simulink model "SwitchMobility_ACC"  (R2022b)
settings: Solver=ode1  StartTime=0.0  StopTime=inf  FixedStep=0.001  RelTol=1e-3
PreLoadFcn:
  | vehicle = 'Truck'; if ~length(which('cmself')), cmenv; end
  | SwitchMobility_ACC_bus
InitFcn:
  | vehicle = 'Truck'; if ~length(which('cmself')), cmenv; end
  | SwitchMobility_ACC_bus
libraries: CarMaker4SL x32, simulink x1
Description:
  | CarMaker Plug-in Model Target
settings Model: Creator=satyaprakash.gupta  LastModifiedBy=satyaprakash.gupta
settings RTWCC: Description=CarMaker Plug-in Model Target  SystemTargetFile=CarMaker.tlc  TemplateMakefile=CarMaker_unix-win64.tmf
settings CodeAppCC: MaxIdLength=127
settings STFCustomTargetCC: TargetLangStandard=C99 (ISO)  CombineOutputUpdateFcns=on  CodeInterfacePackaging=Reusable function  GenerateAllocFcn=on  SystemTargetFile=CarMaker.tlc
settings GRTTargetCC: ParMdlRefBuildCompliant=off  CompOptLevelCompliant=off  ConcurrentExecutionCompliant=off  MatFileLogging=off  CodeInterfacePackaging=Reusable function  CPPClassGenCompliant=off  GenerateAllocFcn=on  UseToolchainInfoCompliant=off

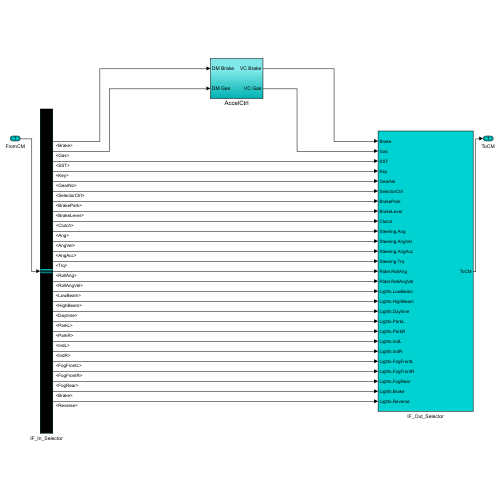
[thumbnail: Simulink's stored preview of the top-level diagram]
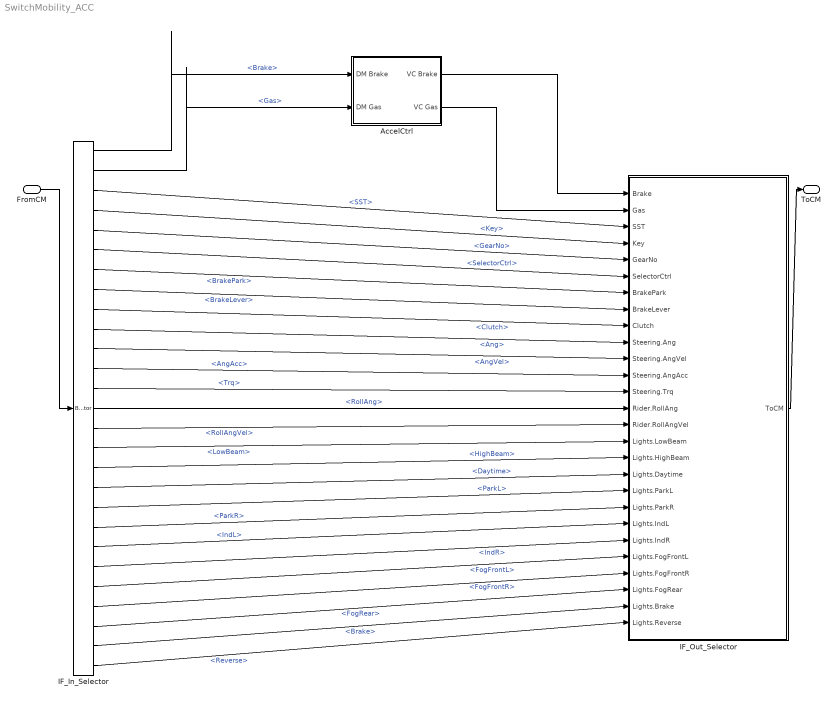
== system SwitchMobility_ACC ==
  FromCM : Inport  OutDataTypeStr=Bus: cmVehicleControlIn
  AccelCtrl : Subsystem
  IF_In_Selector : BusSelector  OutputSignals=Brake,Gas,SST,Key,GearNo,SelectorCtrl,BrakePark,BrakeLever,Clutch,Steering.Ang,Steering.AngVel,Steering.AngAcc,Steering.Trq,Rider.RollAng,Rider.RollAngVel,Lights.LowBeam,Lights.HighBeam,Lights.Daytime,Lights.ParkL,Lights.ParkR,Lights.IndL,Lights.IndR,Lights.FogFrontL,Lights.FogFrontR,Lights.FogRear,Lights.Brake,Lights.Reverse
  IF_Out_Selector : Subsystem  mask(Signal Selection){}
      mask help: Signal Selection Block
      settings: OpenFcn=cmSignalSelect('SignalSelection_CB',gcb)
  ToCM : Outport  OutDataTypeStr=Bus: cmVehicleControlOut
  wires:
  FromCM/1 -> IF_In_Selector/1
  IF_In_Selector/1 -> AccelCtrl/1(DM Brake)  "<Brake>"
  IF_Out_Selector/1(ToCM) -> ToCM/1
  AccelCtrl/1(VC Brake) -> IF_Out_Selector/1(Brake)
  AccelCtrl/2(VC Gas) -> IF_Out_Selector/2(Gas)
  IF_In_Selector/2 -> AccelCtrl/2(DM Gas)  "<Gas>"
  IF_In_Selector/3 -> IF_Out_Selector/3(SST)  "<SST>"
  IF_In_Selector/4 -> IF_Out_Selector/4(Key)  "<Key>"
  IF_In_Selector/5 -> IF_Out_Selector/5(GearNo)  "<GearNo>"
  IF_In_Selector/6 -> IF_Out_Selector/6(SelectorCtrl)  "<SelectorCtrl>"
  IF_In_Selector/7 -> IF_Out_Selector/7(BrakePark)  "<BrakePark>"
  IF_In_Selector/8 -> IF_Out_Selector/8(BrakeLever)  "<BrakeLever>"
  IF_In_Selector/9 -> IF_Out_Selector/9(Clutch)  "<Clutch>"
  IF_In_Selector/10 -> IF_Out_Selector/10(Steering.Ang)  "<Ang>"
  IF_In_Selector/11 -> IF_Out_Selector/11(Steering.AngVel)  "<AngVel>"
  IF_In_Selector/12 -> IF_Out_Selector/12(Steering.AngAcc)  "<AngAcc>"
  IF_In_Selector/13 -> IF_Out_Selector/13(Steering.Trq)  "<Trq>"
  IF_In_Selector/14 -> IF_Out_Selector/14(Rider.RollAng)  "<RollAng>"
  IF_In_Selector/15 -> IF_Out_Selector/15(Rider.RollAngVel)  "<RollAngVel>"
  IF_In_Selector/16 -> IF_Out_Selector/16(Lights.LowBeam)  "<LowBeam>"
  IF_In_Selector/17 -> IF_Out_Selector/17(Lights.HighBeam)  "<HighBeam>"
  IF_In_Selector/18 -> IF_Out_Selector/18(Lights.Daytime)  "<Daytime>"
  IF_In_Selector/19 -> IF_Out_Selector/19(Lights.ParkL)  "<ParkL>"
  IF_In_Selector/20 -> IF_Out_Selector/20(Lights.ParkR)  "<ParkR>"
  IF_In_Selector/21 -> IF_Out_Selector/21(Lights.IndL)  "<IndL>"
  IF_In_Selector/22 -> IF_Out_Selector/22(Lights.IndR)  "<IndR>"
  IF_In_Selector/23 -> IF_Out_Selector/23(Lights.FogFrontL)  "<FogFrontL>"
  IF_In_Selector/24 -> IF_Out_Selector/24(Lights.FogFrontR)  "<FogFrontR>"
  IF_In_Selector/25 -> IF_Out_Selector/25(Lights.FogRear)  "<FogRear>"
  IF_In_Selector/26 -> IF_Out_Selector/26(Lights.Brake)  "<Brake>"
  IF_In_Selector/27 -> IF_Out_Selector/27(Lights.Reverse)  "<Reverse>"

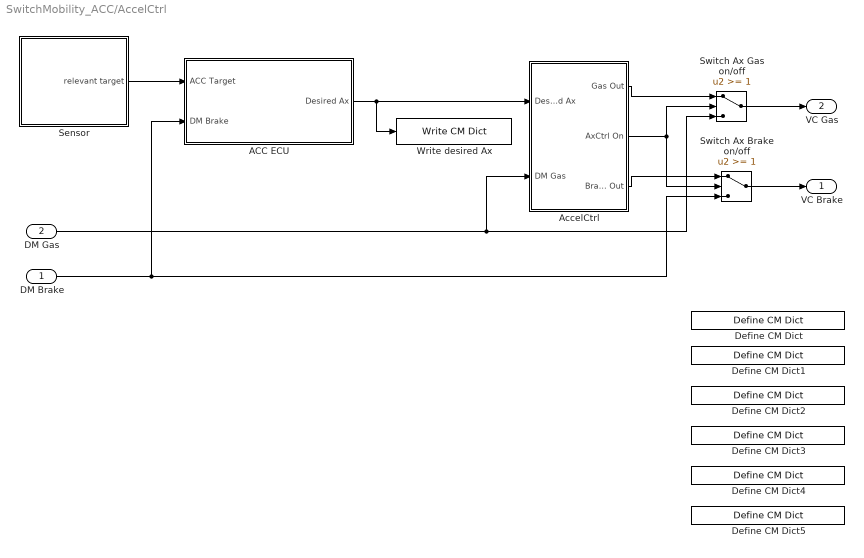
== system SwitchMobility_ACC/AccelCtrl ==
  DM Brake : Inport
  DM Gas : Inport  Port=2
  ACC ECU : Subsystem
  AccelCtrl : Subsystem
  Define CM Dict : CarMaker4SL/Define CM Dict  xname=AccelCtrl.ACC.IsActive  xmono=off  xtype=Char  xdvaplace=DM  xnstates=2  xfirststate=0  xinitial=1
  Define CM Dict1 : CarMaker4SL/Define CM Dict  xname=AccelCtrl.ACC.DesiredTGap  xunit=s  xmono=off  xtype=Double4  xdvaplace=DM  xnstates=0  xfirststate=0  xinitial=0
  Define CM Dict2 : CarMaker4SL/Define CM Dict  xname=AccelCtrl.ACC.DesiredSpd  xunit=m/s  xmono=off  xtype=Double4  xdvaplace=DM  xnstates=0  xfirststate=0  xinitial=0
  Define CM Dict3 : CarMaker4SL/Define CM Dict  xname=AccelCtrl.ACC.DesiredAx  xunit=m/s^2  xmono=off  xtype=Double4  xdvaplace=DM  xnstates=0  xfirststate=0  xinitial=0
  Define CM Dict4 : CarMaker4SL/Define CM Dict  xname=AccelCtrl.DesiredAx  xunit=m/s^2  xmono=off  xtype=Double4  xdvaplace=DM  xnstates=0  xfirststate=0  xinitial=0
  Define CM Dict5 : CarMaker4SL/Define CM Dict  xname=AccelCtrl.ACC.DesiredDist  xunit=m  xmono=off  xtype=Double4  xdvaplace=DM  xnstates=0  xfirststate=0  xinitial=0
  Sensor : Subsystem
  Switch Ax Brake on/off : Switch  Threshold=1  InputSameDT=off
  Switch Ax Gas on/off : Switch  Threshold=1  InputSameDT=off
  Write desired Ax : CarMaker4SL/Write CM Dict  xname=AccelCtrl.DesiredAx  xsync=off
  VC Brake : Outport  VectorParamsAs1DForOutWhenUnconnected=off
  VC Gas : Outport  Port=2  VectorParamsAs1DForOutWhenUnconnected=off
  wires:
  Sensor/1(relevant target) -> ACC ECU/1(ACC Target)
  DM Brake/1 -> Switch Ax Brake on/off/3, ACC ECU/2(DM Brake)
  Switch Ax Gas on/off/1 -> VC Gas/1
  Switch Ax Brake on/off/1 -> VC Brake/1
  AccelCtrl/1(Gas Out) -> Switch Ax Gas on/off/1
  AccelCtrl/3(Brake Out) -> Switch Ax Brake on/off/1
  ACC ECU/1(Desired Ax) -> AccelCtrl/1(Desired Ax), Write desired Ax/1
  DM Gas/1 -> Switch Ax Gas on/off/3, AccelCtrl/2(DM Gas)
  AccelCtrl/2(AxCtrl On) -> Switch Ax Gas on/off/2, Switch Ax Brake on/off/2

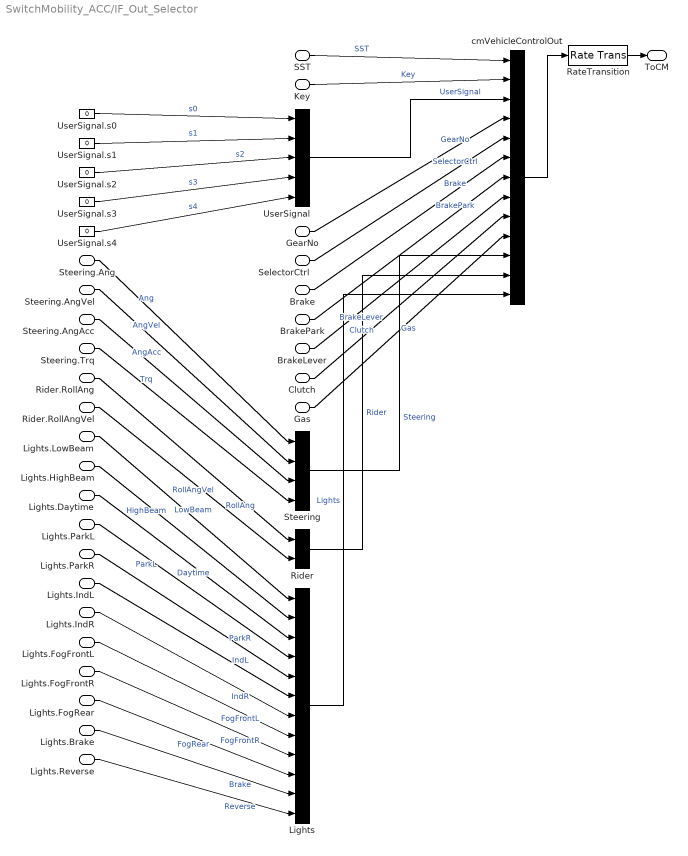
== system SwitchMobility_ACC/IF_Out_Selector ==
  Brake : Inport
  Gas : Inport  Port=2
  SST : Inport  Port=3
  Key : Inport  Port=4
  GearNo : Inport  Port=5
  SelectorCtrl : Inport  Port=6
  BrakePark : Inport  Port=7
  BrakeLever : Inport  Port=8
  Clutch : Inport  Port=9
  Steering.Ang : Inport  Port=10
  Steering.AngVel : Inport  Port=11
  Steering.AngAcc : Inport  Port=12
  Steering.Trq : Inport  Port=13
  Rider.RollAng : Inport  Port=14
  Rider.RollAngVel : Inport  Port=15
  Lights.LowBeam : Inport  Port=16
  Lights.HighBeam : Inport  Port=17
  Lights.Daytime : Inport  Port=18
  Lights.ParkL : Inport  Port=19
  Lights.ParkR : Inport  Port=20
  Lights.IndL : Inport  Port=21
  Lights.IndR : Inport  Port=22
  Lights.FogFrontL : Inport  Port=23
  Lights.FogFrontR : Inport  Port=24
  Lights.FogRear : Inport  Port=25
  Lights.Brake : Inport  Port=26
  Lights.Reverse : Inport  Port=27
  Lights : BusCreator  Inputs=12
  RateTransition : RateTransition  OutPortSampleTime=str2num(get_param(bdroot,'FixedStep'))
  Rider : BusCreator  Inputs=2
  Steering : BusCreator  Inputs=4
  UserSignal : BusCreator  Inputs=5
  UserSignal.s{0..4} (5 alike) : Constant  Value=0
  cmVehicleControlOut : BusCreator  Inputs=13
  ToCM : Outport
  wires:
  RateTransition/1 -> ToCM/1
  cmVehicleControlOut/1 -> RateTransition/1
  UserSignal/1 -> cmVehicleControlOut/3  "UserSignal"
  UserSignal.s0/1 -> UserSignal/1  "s0"
  UserSignal.s1/1 -> UserSignal/2  "s1"
  UserSignal.s2/1 -> UserSignal/3  "s2"
  UserSignal.s3/1 -> UserSignal/4  "s3"
  UserSignal.s4/1 -> UserSignal/5  "s4"
  Steering/1 -> cmVehicleControlOut/11  "Steering"
  Rider/1 -> cmVehicleControlOut/12  "Rider"
  Lights/1 -> cmVehicleControlOut/13  "Lights"
  Brake/1 -> cmVehicleControlOut/6  "Brake"
  Gas/1 -> cmVehicleControlOut/10  "Gas"
  SST/1 -> cmVehicleControlOut/1  "SST"
  Key/1 -> cmVehicleControlOut/2  "Key"
  GearNo/1 -> cmVehicleControlOut/4  "GearNo"
  SelectorCtrl/1 -> cmVehicleControlOut/5  "SelectorCtrl"
  BrakePark/1 -> cmVehicleControlOut/7  "BrakePark"
  BrakeLever/1 -> cmVehicleControlOut/8  "BrakeLever"
  Clutch/1 -> cmVehicleControlOut/9  "Clutch"
  Steering.Ang/1 -> Steering/1  "Ang"
  Steering.AngVel/1 -> Steering/2  "AngVel"
  Steering.AngAcc/1 -> Steering/3  "AngAcc"
  Steering.Trq/1 -> Steering/4  "Trq"
  Rider.RollAng/1 -> Rider/1  "RollAng"
  Rider.RollAngVel/1 -> Rider/2  "RollAngVel"
  Lights.LowBeam/1 -> Lights/1  "LowBeam"
  Lights.HighBeam/1 -> Lights/2  "HighBeam"
  Lights.Daytime/1 -> Lights/3  "Daytime"
  Lights.ParkL/1 -> Lights/4  "ParkL"
  Lights.ParkR/1 -> Lights/5  "ParkR"
  Lights.IndL/1 -> Lights/6  "IndL"
  Lights.IndR/1 -> Lights/7  "IndR"
  Lights.FogFrontL/1 -> Lights/8  "FogFrontL"
  Lights.FogFrontR/1 -> Lights/9  "FogFrontR"
  Lights.FogRear/1 -> Lights/10  "FogRear"
  Lights.Brake/1 -> Lights/11  "Brake"
  Lights.Reverse/1 -> Lights/12  "Reverse"

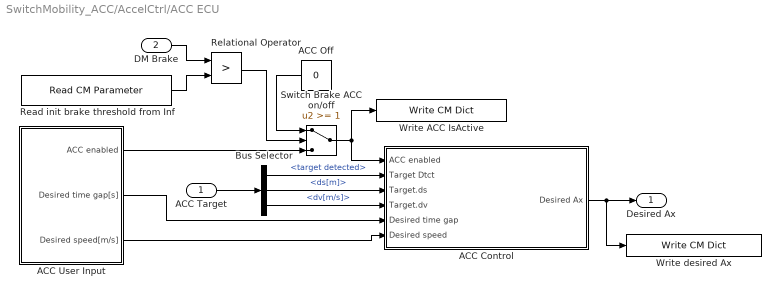
== system SwitchMobility_ACC/AccelCtrl/ACC ECU ==
  ACC Target : Inport
  DM Brake : Inport  Port=2
  ACC Control : Subsystem
  ACC Off : Constant  Value=0
  ACC User Input : Subsystem
  Bus Selector : BusSelector  OutputSignals=target detected,ds[m],dv[m/s]
  Read init brake threshold from Inf : CarMaker4SL/Read CM Parameter  xfile=Vehicle  xkey=AccelCtrl.ACC.BrakeThreshold  xnout=1  xdefaults=0.2  xmuxed=off  xstime=Continuous
      settings: SourceProductName=CarMaker4SL
  Relational Operator : RelationalOperator  Operator=>  InputSameDT=off
  Switch Brake ACC on/off : Switch  Threshold=1  InputSameDT=off
  Write ACC IsActive : CarMaker4SL/Write CM Dict  xname=AccelCtrl.ACC.IsActive  xsync=off
  Write desired Ax : CarMaker4SL/Write CM Dict  xname=AccelCtrl.ACC.DesiredAx  xsync=off
  Desired Ax : Outport  VectorParamsAs1DForOutWhenUnconnected=off
  wires:
  ACC Target/1 -> Bus Selector/1
  Bus Selector/2 -> ACC Control/3(Target.ds)  "<ds[m]>"
  Bus Selector/3 -> ACC Control/4(Target.dv)  "<dv[m/s]>"
  Bus Selector/1 -> ACC Control/2(Target Dtct)  "<target detected>"
  ACC Control/1(Desired Ax) -> Desired Ax/1, Write desired Ax/1
  ACC User Input/2(Desired time gap[s]) -> ACC Control/5(Desired time gap)
  ACC User Input/3(Desired speed[m/s]) -> ACC Control/6(Desired speed)
  DM Brake/1 -> Relational Operator/1
  ACC User Input/1(ACC enabled) -> Switch Brake ACC on/off/3
  Relational Operator/1 -> Switch Brake ACC on/off/2
  ACC Off/1 -> Switch Brake ACC on/off/1
  Switch Brake ACC on/off/1 -> ACC Control/1(ACC enabled), Write ACC IsActive/1
  Read init brake threshold from Inf/1 -> Relational Operator/2

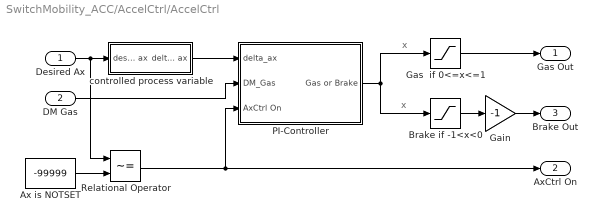
== system SwitchMobility_ACC/AccelCtrl/AccelCtrl ==
  note: x
  note: x
  Desired Ax : Inport
  DM Gas : Inport  Port=2
  Ax is NOTSET : Constant  Value=-99999
  Brake if -1<x<0 : Saturate  UpperLimit=0  LowerLimit=-1
  Gain : Gain  Gain=-1  SaturateOnIntegerOverflow=on  OutDataTypeStr=Inherit: Same as input  ParamDataTypeStr=Inherit: Same as input
  Gas  if 0<=x<=1 : Saturate  UpperLimit=1  LowerLimit=0
  PI-Controller : Subsystem
  Relational Operator : RelationalOperator  Operator=~=  InputSameDT=off
  "controlled process variable " : Subsystem
  Gas Out : Outport  VectorParamsAs1DForOutWhenUnconnected=off
  AxCtrl On : Outport  Port=2  VectorParamsAs1DForOutWhenUnconnected=off
  Brake Out : Outport  Port=3  VectorParamsAs1DForOutWhenUnconnected=off
  wires:
  Gain/1 -> Brake Out/1
  "controlled process variable "/1(delta ax) -> PI-Controller/1(delta_ax)
  DM Gas/1 -> PI-Controller/2(DM_Gas)
  Desired Ax/1 -> "controlled process variable "/1(desired ax), Relational Operator/1
  PI-Controller/1(Gas or Brake) -> Brake if -1<x<0/1, Gas  if 0<=x<=1/1
  Gas  if 0<=x<=1/1 -> Gas Out/1
  Brake if -1<x<0/1 -> Gain/1
  Ax is NOTSET/1 -> Relational Operator/2
  Relational Operator/1 -> AxCtrl On/1, PI-Controller/3(AxCtrl On)

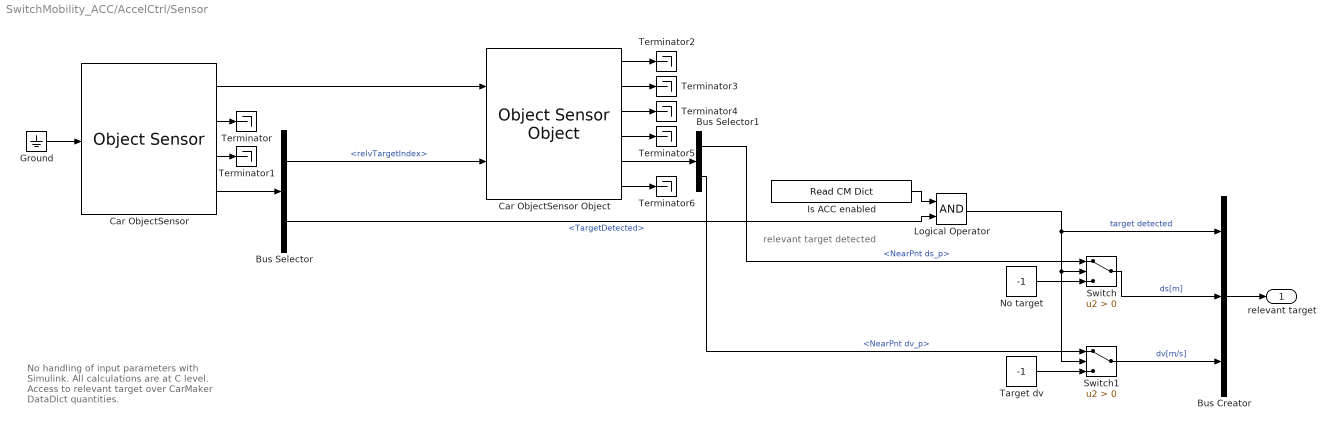
== system SwitchMobility_ACC/AccelCtrl/Sensor ==
  note: No handling of
      | input parameters with Simulink.
      | All calculations are at C level.
      | Access to relevant target
      | over CarMaker DataDict quantities.
  note: relevant target detected
  Bus Creator : BusCreator  Inputs=3
  Bus Selector : BusSelector  OutputSignals=relvTargetIndex,TargetDetected
  Bus Selector1 : BusSelector  OutputSignals=NearPnt ds_p,NearPnt dv_p
  Car ObjectSensor : CarMaker4SL/Sensors/Object Sensor  xname=RadarL  xstime=Continuous
      settings: SourceProductName=CarMaker4SL
  Car ObjectSensor Object : CarMaker4SL/Sensors/Object Sensor Object  xname=INPORT  ximode=World Objects  xstime=Continuous
      settings: SourceProductName=CarMaker4SL
  Ground : Ground
  Is ACC enabled : CarMaker4SL/Read CM Dict  xname=AccelCtrl.ACC.IsActive  xsync=off  xstime=Continuous
  Logical Operator : Logic  AllPortsSameDT=off
  No target : Constant  Value=-1
  Switch : Switch  Criteria=u2 > Threshold  InputSameDT=off
  Switch1 : Switch  Criteria=u2 > Threshold  InputSameDT=off
  Target dv : Constant  Value=-1
  Terminator{,1..6} (7 alike) : Terminator
  relevant target : Outport  VectorParamsAs1DForOutWhenUnconnected=off
  wires:
  Switch/1 -> Bus Creator/2  "ds[m]"
  Bus Selector1/1 -> Switch/1  "<NearPnt ds_p>"
  No target/1 -> Switch/3
  Bus Selector1/2 -> Switch1/1  "<NearPnt dv_p>"
  Target dv/1 -> Switch1/3
  Switch1/1 -> Bus Creator/3  "dv[m/s]"
  Bus Creator/1 -> relevant target/1
  Is ACC enabled/1 -> Logical Operator/1
  Logical Operator/1 -> Bus Creator/1, Switch1/2, Switch/2  "target detected"
  Car ObjectSensor/1 -> Car ObjectSensor Object/1
  Ground/1 -> Car ObjectSensor/1
  Car ObjectSensor/4 -> Bus Selector/1
  Bus Selector/2 -> Logical Operator/2  "<TargetDetected>"
  Bus Selector/1 -> Car ObjectSensor Object/2  "<relvTargetIndex>"
  Car ObjectSensor Object/5 -> Bus Selector1/1
  Car ObjectSensor/2 -> Terminator/1
  Car ObjectSensor/3 -> Terminator1/1
  Car ObjectSensor Object/1 -> Terminator2/1
  Car ObjectSensor Object/2 -> Terminator3/1
  Car ObjectSensor Object/3 -> Terminator4/1
  Car ObjectSensor Object/4 -> Terminator5/1
  Car ObjectSensor Object/6 -> Terminator6/1

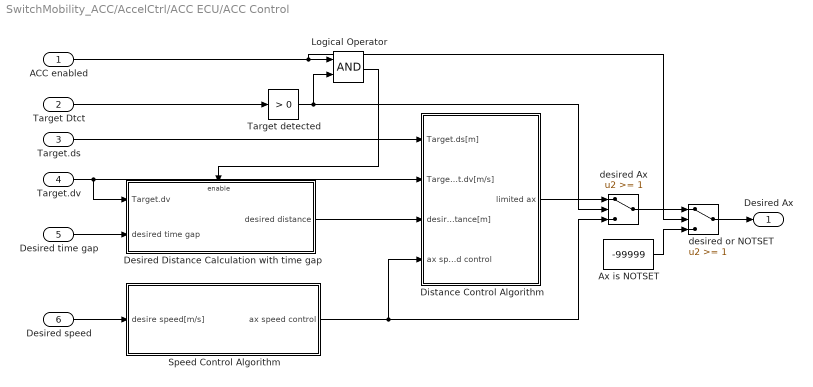
== system SwitchMobility_ACC/AccelCtrl/ACC ECU/ACC Control ==
  ACC enabled : Inport
  Target Dtct : Inport  Port=2
  Target.ds : Inport  Port=3
  Target.dv : Inport  Port=4
  Desired time gap : Inport  Port=5
  Desired speed : Inport  Port=6
  Ax is NOTSET : Constant  Value=-99999
  Desired Distance Calculation with time gap : Subsystem  TreatAsAtomicUnit=on
  Distance Control Algorithm : Subsystem  TreatAsAtomicUnit=on
  Logical Operator : Logic  AllPortsSameDT=off
  Speed Control Algorithm : Subsystem  TreatAsAtomicUnit=on
  Target detected : simulink/Logic and Bit Operations/Compare To Zero  relop=>  OutDataTypeStr=uint8  ZeroCross=off
  desired Ax : Switch  Threshold=1  InputSameDT=off
  desired or NOTSET : Switch  Threshold=1  InputSameDT=off
  Desired Ax : Outport  VectorParamsAs1DForOutWhenUnconnected=off
  wires:
  Target.dv/1 -> Distance Control Algorithm/2(Target.dv[m/s]), Desired Distance Calculation with time gap/1(Target.dv)
  Target.ds/1 -> Distance Control Algorithm/1(Target.ds[m])
  Target Dtct/1 -> Target detected/1
  Distance Control Algorithm/1("  limited ax") -> desired Ax/1
  Target detected/1 -> desired Ax/2, Logical Operator/2
  Desired Distance Calculation with time gap/1(desired distance) -> Distance Control Algorithm/3(desired distance[m])
  Desired time gap/1 -> Desired Distance Calculation with time gap/2(desired time gap)
  Desired speed/1 -> Speed Control Algorithm/1(desire speed[m/s])
  Speed Control Algorithm/1(ax speed control) -> desired Ax/3, Distance Control Algorithm/4(ax speed control)
  ACC enabled/1 -> Logical Operator/1, desired or NOTSET/2
  Logical Operator/1 -> Desired Distance Calculation with time gap/Enable
  desired or NOTSET/1 -> Desired Ax/1
  desired Ax/1 -> desired or NOTSET/1
  Ax is NOTSET/1 -> desired or NOTSET/3

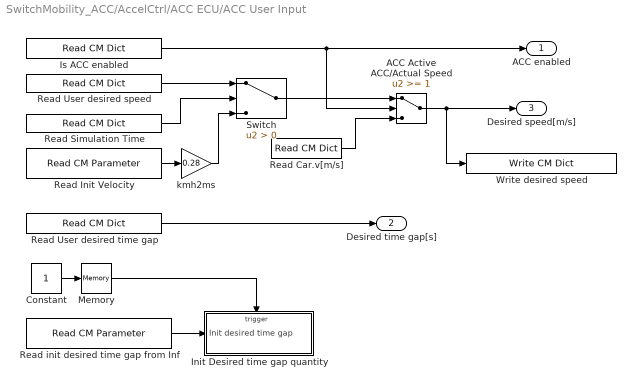
== system SwitchMobility_ACC/AccelCtrl/ACC ECU/ACC User Input ==
  ACC Active ACC/Actual Speed : Switch  Threshold=1  InputSameDT=off
  Constant : Constant
  Init Desired time gap quantity : Subsystem  TreatAsAtomicUnit=on
  Is ACC enabled : CarMaker4SL/Read CM Dict  xname=AccelCtrl.ACC.IsActive  xsync=off  xstime=Continuous
  Memory : Memory
  Read Car.v[m/s] : CarMaker4SL/Read CM Dict  xname=Car.v  xsync=off  xstime=Continuous
  Read Init Velocity : CarMaker4SL/Read CM Parameter  xfile=Testrun  xkey=DrivMan.Man.Start.Velocity  xnout=1  xdefaults=0  xmuxed=on  xstime=Continuous
      settings: SourceProductName=CarMaker4SL
  Read Simulation Time : CarMaker4SL/Read CM Dict  xname=Time  xsync=off  xstime=Continuous
  Read User desired speed : CarMaker4SL/Read CM Dict  xname=AccelCtrl.ACC.DesiredSpd  xsync=off  xstime=Continuous
  Read User desired time gap : CarMaker4SL/Read CM Dict  xname=AccelCtrl.ACC.DesiredTGap  xsync=off  xstime=Continuous
  Read init desired time gap from Inf : CarMaker4SL/Read CM Parameter  xfile=Vehicle  xkey=AccelCtrl.ACC.DesrTGap  xnout=1  xdefaults=1.8  xmuxed=off  xstime=Continuous
      settings: SourceProductName=CarMaker4SL
  Switch : Switch  Criteria=u2 > Threshold  SaturateOnIntegerOverflow=off  InputSameDT=off
  Write desired speed : CarMaker4SL/Write CM Dict  xname=AccelCtrl.ACC.DesiredSpd  xsync=off
  kmh2ms : Gain  Gain=0.28
  ACC enabled : Outport  VectorParamsAs1DForOutWhenUnconnected=off
  Desired time gap[s] : Outport  Port=2  VectorParamsAs1DForOutWhenUnconnected=off
  Desired speed[m/s] : Outport  Port=3  VectorParamsAs1DForOutWhenUnconnected=off
  wires:
  Is ACC enabled/1 -> ACC enabled/1, ACC Active ACC/Actual Speed/2
  Read Car.v[m/s]/1 -> ACC Active ACC/Actual Speed/3
  ACC Active ACC/Actual Speed/1 -> Desired speed[m/s]/1, Write desired speed/1
  Read User desired time gap/1 -> Desired time gap[s]/1
  Constant/1 -> Memory/1
  Memory/1 -> Init Desired time gap quantity/Trigger
  Read init desired time gap from Inf/1 -> Init Desired time gap quantity/1("Init desired time gap ")
  Read Init Velocity/1 -> kmh2ms/1
  Switch/1 -> ACC Active ACC/Actual Speed/1
  Read User desired speed/1 -> Switch/1
  Read Simulation Time/1 -> Switch/2
  kmh2ms/1 -> Switch/3

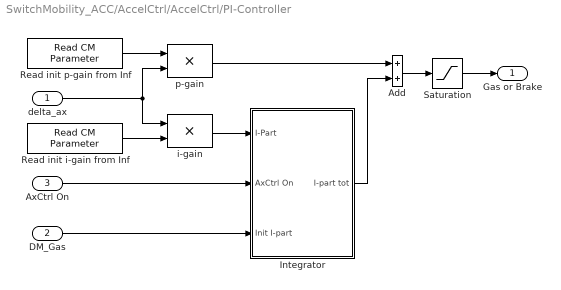
== system SwitchMobility_ACC/AccelCtrl/AccelCtrl/PI-Controller ==
  delta_ax : Inport
  DM_Gas : Inport  Port=2
  AxCtrl On : Inport  Port=3
  Add : Sum  SaturateOnIntegerOverflow=on  OutDataTypeStr=Inherit: Same as first input
  Integrator : Subsystem
  Read init i-gain from Inf : CarMaker4SL/Read CM Parameter  xfile=Vehicle  xkey=AccelCtrl.i  xnout=1  xdefaults=0.001  xmuxed=off  xstime=Continuous
      settings: SourceProductName=CarMaker4SL
  Read init p-gain from Inf : CarMaker4SL/Read CM Parameter  xfile=Vehicle  xkey=AccelCtrl.p  xnout=1  xdefaults=0.001  xmuxed=off  xstime=Continuous
      settings: SourceProductName=CarMaker4SL
  Saturation : Saturate  UpperLimit=1  LowerLimit=-1
  i-gain : Product  SaturateOnIntegerOverflow=on  OutDataTypeStr=Inherit: Same as first input
  p-gain : Product  SaturateOnIntegerOverflow=on  OutDataTypeStr=Inherit: Same as first input
  Gas or Brake : Outport  VectorParamsAs1DForOutWhenUnconnected=off
  wires:
  Saturation/1 -> Gas or Brake/1
  Add/1 -> Saturation/1
  p-gain/1 -> Add/1
  delta_ax/1 -> p-gain/2, i-gain/1
  i-gain/1 -> Integrator/1(I-Part)
  AxCtrl On/1 -> Integrator/2(AxCtrl On)
  DM_Gas/1 -> Integrator/3(Init I-part)
  Integrator/1("I-part tot ") -> Add/2
  Read init p-gain from Inf/1 -> p-gain/1
  Read init i-gain from Inf/1 -> i-gain/2

== system SwitchMobility_ACC/AccelCtrl/AccelCtrl/controlled process variable  ==
  desired ax : Inport
  Read Car.ax : CarMaker4SL/Read CM Dict  xname=Car.ax  xsync=off  xstime=Continuous
  Subtract : Sum  Inputs=+-  SaturateOnIntegerOverflow=on
  delta ax : Outport  VectorParamsAs1DForOutWhenUnconnected=off
  wires:
  desired ax/1 -> Subtract/1
  Read Car.ax/1 -> Subtract/2
  Subtract/1 -> delta ax/1

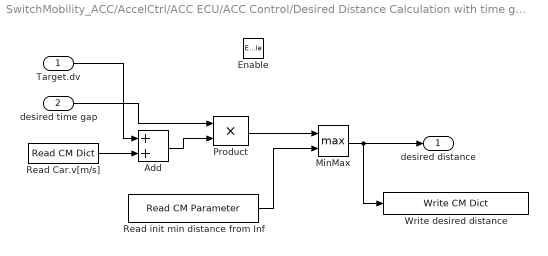
== system SwitchMobility_ACC/AccelCtrl/ACC ECU/ACC Control/Desired Distance Calculation with time gap ==
  Target.dv : Inport
  desired time gap : Inport  Port=2
  Enable : EnablePort
  Add : Sum  SaturateOnIntegerOverflow=on  OutDataTypeStr=Inherit: Same as first input
  MinMax : MinMax  Function=max  Inputs=2  InputSameDT=on  SaturateOnIntegerOverflow=on
  Product : Product  SaturateOnIntegerOverflow=on  OutDataTypeStr=Inherit: Same as first input
  Read Car.v[m/s] : CarMaker4SL/Read CM Dict  xname=Car.v  xsync=off  xstime=Continuous
  Read init min distance from Inf : CarMaker4SL/Read CM Parameter  xfile=Vehicle  xkey=AccelCtrl.ACC.DistMin  xnout=1  xdefaults=20  xmuxed=off  xstime=Continuous
      settings: SourceProductName=CarMaker4SL
  Write desired distance : CarMaker4SL/Write CM Dict  xname=AccelCtrl.ACC.DesiredDist  xsync=off
  desired distance : Outport  InitialOutput=0  VectorParamsAs1DForOutWhenUnconnected=off
  wires:
  Read Car.v[m/s]/1 -> Add/2
  Product/1 -> MinMax/1
  Add/1 -> Product/2
  desired time gap/1 -> Product/1
  Target.dv/1 -> Add/1
  MinMax/1 -> desired distance/1, Write desired distance/1
  Read init min distance from Inf/1 -> MinMax/2

== system SwitchMobility_ACC/AccelCtrl/ACC ECU/ACC Control/Distance Control Algorithm ==
  Target.ds[m] : Inport
  Target.dv[m/s] : Inport  Port=2
  desired distance[m] : Inport  Port=3
  ax speed control : Inport  Port=4
  -2.5<=ax<=1 : Saturate  UpperLimit=1  LowerLimit=-2.5
  desired ax : Subsystem
  "  limited ax" : Outport  InitialOutput=0  VectorParamsAs1DForOutWhenUnconnected=off
  wires:
  ax speed control/1 -> desired ax/4(ax speed control)
  desired distance[m]/1 -> desired ax/3(desired distance[m])
  Target.dv[m/s]/1 -> desired ax/2(Target.dv[m/s])
  Target.ds[m]/1 -> desired ax/1(Target.ds[m])
  -2.5<=ax<=1/1 -> "  limited ax"/1
  desired ax/1(desired ax) -> -2.5<=ax<=1/1

== system SwitchMobility_ACC/AccelCtrl/ACC ECU/ACC Control/Speed Control Algorithm ==
  desire speed[m/s] : Inport
  -0.35<=ax<=1 : Saturate  UpperLimit=1  LowerLimit=-0.35
  desired ax : Subsystem
  ax speed control : Outport  InitialOutput=0  VectorParamsAs1DForOutWhenUnconnected=off
  wires:
  desire speed[m/s]/1 -> desired ax/1(desire speed[m/s])
  desired ax/1(desired ax) -> -0.35<=ax<=1/1
  -0.35<=ax<=1/1 -> ax speed control/1

== system SwitchMobility_ACC/AccelCtrl/ACC ECU/ACC User Input/Init Desired time gap quantity ==
  "Init desired time gap " : Inport
  Trigger : TriggerPort  VariantControl=Variant
  Write init time gap : CarMaker4SL/Write CM Dict  xname=AccelCtrl.ACC.DesiredTGap  xsync=off
  wires:
  "Init desired time gap "/1 -> Write init time gap/1

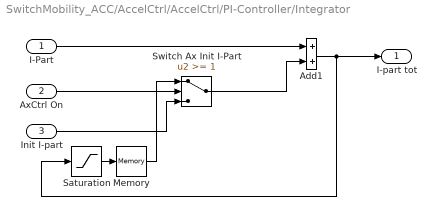
== system SwitchMobility_ACC/AccelCtrl/AccelCtrl/PI-Controller/Integrator ==
  I-Part : Inport
  AxCtrl On : Inport  Port=2
  Init I-part : Inport  Port=3
  Add1 : Sum  SaturateOnIntegerOverflow=on  OutDataTypeStr=Inherit: Same as first input
  Memory : Memory
  Saturation : Saturate  UpperLimit=1  LowerLimit=-1
  Switch Ax Init I-Part : Switch  Threshold=1  InputSameDT=off
  "I-part tot " : Outport  VectorParamsAs1DForOutWhenUnconnected=off
  wires:
  Saturation/1 -> Memory/1
  Switch Ax Init I-Part/1 -> Add1/2
  Add1/1 -> Saturation/1, "I-part tot "/1
  I-Part/1 -> Add1/1
  AxCtrl On/1 -> Switch Ax Init I-Part/2
  Memory/1 -> Switch Ax Init I-Part/1
  Init I-part/1 -> Switch Ax Init I-Part/3

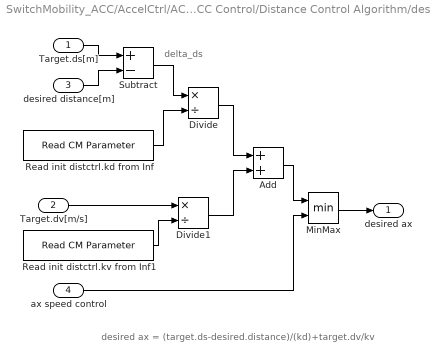
== system SwitchMobility_ACC/AccelCtrl/ACC ECU/ACC Control/Distance Control Algorithm/desired ax ==
  note: desired ax = (target.ds-desired.distance)/(kd)+target.dv/kv
  note: delta_ds
  Target.ds[m] : Inport
  Target.dv[m/s] : Inport  Port=2
  desired distance[m] : Inport  Port=3
  ax speed control : Inport  Port=4
  Add : Sum  SaturateOnIntegerOverflow=on  OutDataTypeStr=Inherit: Same as first input
  Divide : Product  Inputs=*/  SaturateOnIntegerOverflow=on  OutDataTypeStr=Inherit: Same as first input
  Divide1 : Product  Inputs=*/  SaturateOnIntegerOverflow=on  OutDataTypeStr=Inherit: Same as first input
  MinMax : MinMax  Inputs=2  InputSameDT=on  SaturateOnIntegerOverflow=on
  Read init distctrl.kd from Inf : CarMaker4SL/Read CM Parameter  xfile=Vehicle  xkey=AccelCtrl.ACC.DistCtrl.kd  xnout=1  xdefaults=36  xmuxed=off  xstime=Continuous
      settings: SourceProductName=CarMaker4SL
  Read init distctrl.kv from Inf1 : CarMaker4SL/Read CM Parameter  xfile=Vehicle  xkey=AccelCtrl.ACC.DistCtrl.kv  xnout=1  xdefaults=2  xmuxed=off  xstime=Continuous
      settings: SourceProductName=CarMaker4SL
  Subtract : Sum  Inputs=+-  SaturateOnIntegerOverflow=on  OutDataTypeStr=Inherit: Same as first input
  desired ax : Outport  VectorParamsAs1DForOutWhenUnconnected=off
  wires:
  MinMax/1 -> desired ax/1
  ax speed control/1 -> MinMax/2
  Add/1 -> MinMax/1
  Divide1/1 -> Add/2
  Divide/1 -> Add/1
  Subtract/1 -> Divide/1
  desired distance[m]/1 -> Subtract/2
  Target.ds[m]/1 -> Subtract/1
  Target.dv[m/s]/1 -> Divide1/1
  Read init distctrl.kd from Inf/1 -> Divide/2
  Read init distctrl.kv from Inf1/1 -> Divide1/2

== system SwitchMobility_ACC/AccelCtrl/ACC ECU/ACC Control/Speed Control Algorithm/desired ax ==
  desire speed[m/s] : Inport
  Divide : Product  Inputs=*/  SaturateOnIntegerOverflow=on  OutDataTypeStr=Inherit: Same as first input
  Read Car.v[m/s] : CarMaker4SL/Read CM Dict  xname=Car.v  xsync=off  xstime=Continuous
  Read init spdctrl.kv from Inf : CarMaker4SL/Read CM Parameter  xfile=Vehicle  xkey=AccelCtrl.ACC.SpdCtrl.kv  xnout=1  xdefaults=13  xmuxed=off  xstime=Continuous
      settings: SourceProductName=CarMaker4SL
  Sum : Sum  Inputs=|+-  SaturateOnIntegerOverflow=on  OutDataTypeStr=Inherit: Same as first input
  desired ax : Outport  VectorParamsAs1DForOutWhenUnconnected=off
  wires:
  Divide/1 -> desired ax/1
  desire speed[m/s]/1 -> Sum/1
  Read Car.v[m/s]/1 -> Sum/2
  Sum/1 -> Divide/1
  Read init spdctrl.kv from Inf/1 -> Divide/2
